simulink model "mositure_Sensor_control"  (R2023a)
settings: Solver=FixedStepAuto  StartTime=0.0  StopTime=inf  FixedStep=0.001  RelTol=1e-3
values from neighbouring files (symbols this model uses):
  K = 5    [mositure_Sensor.m]
settings Model: Creator=alaam  LastModifiedBy=alaam
settings OptimizationCC: DefaultParameterBehavior=Inlined  UseDivisionForNetSlopeComputation=on  GainParamInheritBuiltInType=on  UseFloatMulNetSlope=on  InlineInvariantSignals=on  PassReuseOutputArgsAs=Individual arguments  ZeroExternalMemoryAtStartup=off  ZeroInternalMemoryAtStartup=off  NoFixptDivByZeroProtection=on  EfficientFloat2IntCast=on  LifeSpan=1  OptimizeBlockOrder=speed  DifferentSizesBufferReuse=on  EfficientTunableParamExpr=on
settings DebuggingCC: ParameterTunabilityLossMsg=error
settings HardwareCC: ProdBitPerInt=16  ProdBitPerPointer=16  ProdBitPerSizeT=16  ProdBitPerPtrDiffT=16  ProdLargestAtomicFloat=None  ProdWordSize=8  ProdLongLongMode=on  ProdHWDeviceType=Atmel->AVR
settings SFSimCC: MATLABDynamicMemAlloc=off
settings RTWCC: Description=Embedded Coder  SystemTargetFile=ert.tlc  TemplateMakefile=ert_default_tmf
settings CodeAppCC: ForceParamTrailComments=on  IgnoreCustomStorageClasses=off  OperatorAnnotations=on  SimulinkDataObjDesc=on  SFDataObjDesc=on  CustomSymbolStrGlobalVar=rt$N$M  CustomSymbolStrType=$N$M  CustomSymbolStrFcn=$N$M$F  CustomSymbolStrMacro=$N$M  InsertBlockDesc=on
settings ERTTargetCC: TargetLangStandard=C99 (ISO)  GenerateSampleERTMain=on  IncludeMdlTerminateFcn=off  CombineSignalStateStructs=on  SupportComplex=off  SupportContinuousTime=on  InlinedParameterPlacement=NonHierarchical  ERTCustomFileTemplate=example_file_process.tlc  ERTFilePackagingFormat=CompactWithDataFile

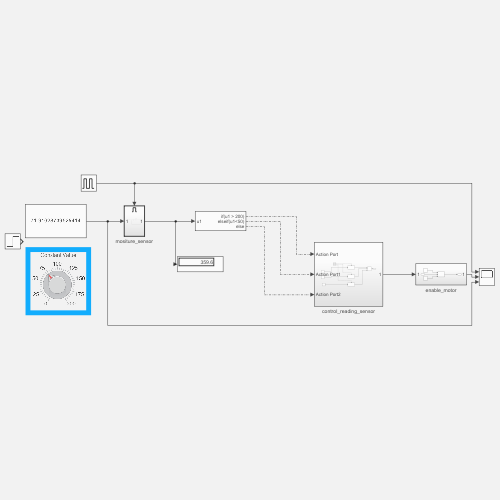
[thumbnail: Simulink's stored preview of the top-level diagram]
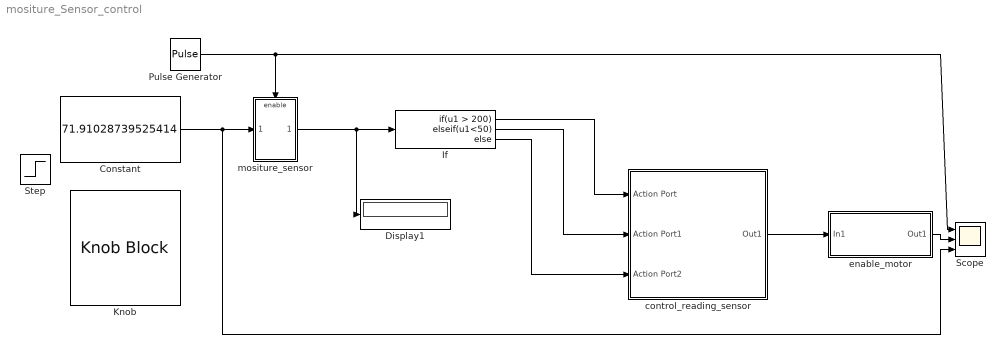
== system mositure_Sensor_control ==
  Constant : Constant  Value=71.91028739525414
  Display1 : Display
  If : If  IfExpression=u1 > 200  ElseIfExpressions=u1<50
  Knob : KnobBlock  ScaleMax=200
  Pulse Generator : DiscretePulseGenerator  PulseType=Time based  Period=10  PulseWidth=50
  Scope : Scope  NumInputPorts=3
  Step : Step  SampleTime=0
  control_reading_sensor : Subsystem
  enable_motor : Subsystem
  mositure_sensor : Subsystem
  wires:
  If/1 -> control_reading_sensor/1(Action Port)
  If/2 -> control_reading_sensor/2(Action Port1)
  If/3 -> control_reading_sensor/3(Action Port2)
  mositure_sensor/1(Out1) -> Display1/1, If/1
  Constant/1 -> Scope/3, mositure_sensor/1(Input)
  control_reading_sensor/1(Out1) -> enable_motor/1(In1)
  enable_motor/1(Out1) -> Scope/2
  Pulse Generator/1 -> Scope/1, mositure_sensor/Enable

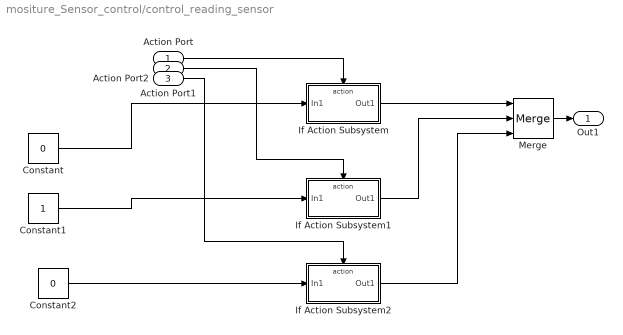
== system mositure_Sensor_control/control_reading_sensor ==
  Action Port : Inport
  Action Port1 : Inport  Port=2
  Action Port2 : Inport  Port=3
  Constant : Constant  Value=0
  Constant1 : Constant
  Constant2 : Constant  Value=0
  If Action Subsystem : Subsystem  TreatAsAtomicUnit=on
  If Action Subsystem1 : Subsystem  TreatAsAtomicUnit=on
  If Action Subsystem2 : Subsystem  TreatAsAtomicUnit=on
  Merge : Merge  Inputs=3
  Out1 : Outport
  wires:
  If Action Subsystem2/1(Out1) -> Merge/3
  If Action Subsystem1/1(Out1) -> Merge/2
  Merge/1 -> Out1/1
  If Action Subsystem/1(Out1) -> Merge/1
  Action Port1/1 -> If Action Subsystem1/Action
  Action Port/1 -> If Action Subsystem/Action
  Action Port2/1 -> If Action Subsystem2/Action
  Constant/1 -> If Action Subsystem/1(In1)
  Constant2/1 -> If Action Subsystem2/1(In1)
  Constant1/1 -> If Action Subsystem1/1(In1)

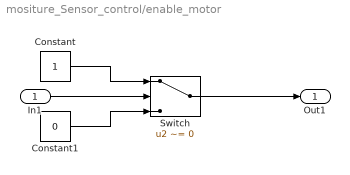
== system mositure_Sensor_control/enable_motor ==
  In1 : Inport
  Constant : Constant
  Constant1 : Constant  Value=0
  Switch : Switch  Criteria=u2 ~= 0  SaturateOnIntegerOverflow=off  InputSameDT=off
  Out1 : Outport
  wires:
  In1/1 -> Switch/2
  Constant/1 -> Switch/1
  Constant1/1 -> Switch/3
  Switch/1 -> Out1/1

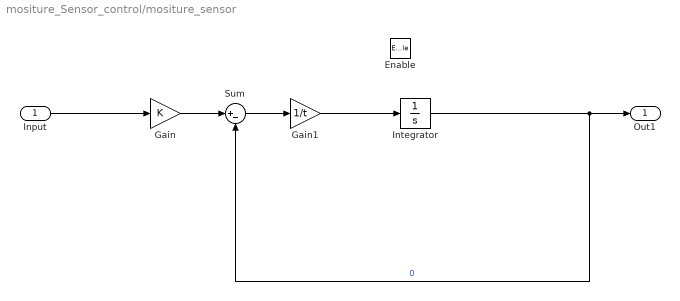
== system mositure_Sensor_control/mositure_sensor ==
  Input : Inport
  Enable : EnablePort
  Gain : Gain  Gain=K
  Gain1 : Gain  Gain=1/t
  Integrator : Integrator
  Sum : Sum  Inputs=|+-
  Out1 : Outport
  wires:
  Sum/1 -> Gain1/1
  Integrator/1 -> Out1/1, Sum/2  "0"
  Gain1/1 -> Integrator/1
  Input/1 -> Gain/1
  Gain/1 -> Sum/1

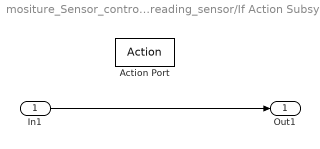
== system mositure_Sensor_control/control_reading_sensor/If Action Subsystem ==
  In1 : Inport
  Action Port : ActionPort  ActionPortLabel=if(u1 > 200)
  Out1 : Outport
  wires:
  In1/1 -> Out1/1

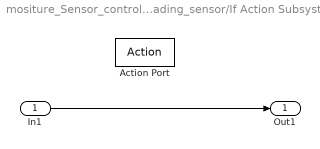
== system mositure_Sensor_control/control_reading_sensor/If Action Subsystem1 ==
  In1 : Inport
  Action Port : ActionPort  ActionPortLabel=elseif(u1<50)
  Out1 : Outport
  wires:
  In1/1 -> Out1/1

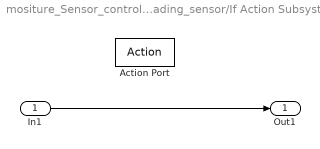
== system mositure_Sensor_control/control_reading_sensor/If Action Subsystem2 ==
  In1 : Inport
  Action Port : ActionPort  ActionPortLabel=else
  Out1 : Outport
  wires:
  In1/1 -> Out1/1
